simulink model "LocalTerrain"  (R2024a)
settings: configuration reference "standardSILConfiguraitonParams" (kept outside this file)
undefined symbols (not defined in the file): terrainHeightNED_m
settings Model: Creator=jerem  LastModifiedBy=jerem
settings ConfigSetRef: SourceName=standardSILConfiguraitonParams  SourceLocation=Base Workspace

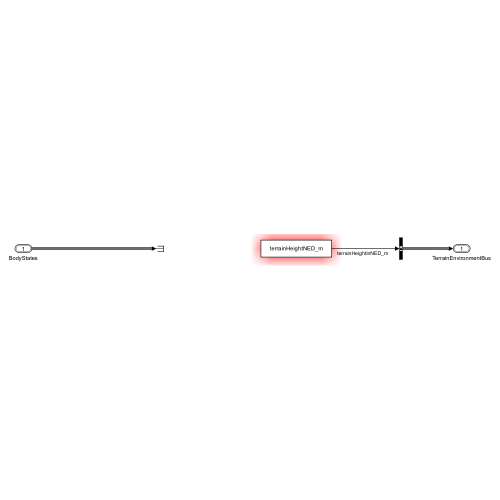
[thumbnail: Simulink's stored preview of the top-level diagram]
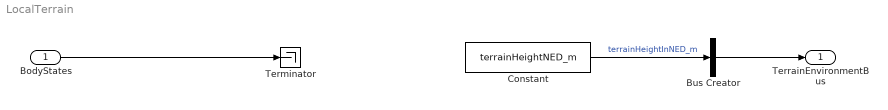
== system LocalTerrain ==
  BodyStates : Inport  OutDataTypeStr=Bus: BodyStateBus
  Bus Creator : BusCreator  Inputs=1  OutDataTypeStr=Bus: TerrainEnvironmentBus
  Constant : Constant  Value=terrainHeightNED_m
  Terminator : Terminator
  TerrainEnvironmentBus : Outport  OutDataTypeStr=Bus: TerrainEnvironmentBus
  wires:
  BodyStates/1 -> Terminator/1
  Constant/1 -> Bus Creator/1  "terrainHeightInNED_m"
  Bus Creator/1 -> TerrainEnvironmentBus/1
